simulink model "TCSC_original"  (R2024a)
settings: Solver=FixedStepAuto  StartTime=0.0  StopTime=5  FixedStep=Ts  MaxStep=2*Ts  RelTol=1e-4  AbsTol=1e-4
PreLoadFcn:
  | Ts=50e-6;
undefined symbols (not defined in the file or in its folder): DiscIntNeverNeededParam, find_system
libraries: spsEdgeDetectorLib x12, spsSampleandHoldLib x6, spsSeriesRLCBranchLib x6, spsThyristorLib x6, spsVoltageMeasurementLib x4, spsBistableLib x3, spsMeanVariableFrequencyLib x3, spsSecondOrderFilterLib x3, spsBreakerLib x3, spsCurrentMeasurementLib x3, spsThreePhaseVIMeasurementLib x2, spsGroundLib x2
(part 1 of 2)
settings Model: Creator=The MathWorks, Inc.  LastModifiedBy=E370_
settings SolverCC: AutoScaleAbsTol=off  AlgebraicLoopSolver=TrustRegion
settings DataIOCC: SaveFormat=StructureWithTime  SaveOutput=off  SignalLogging=off  DSMLogging=off  SaveTime=off  ReturnWorkspaceOutputs=off  SignalLoggingName=sigsOut
settings OptimizationCC: BooleanDataType=off  ExpressionDepthLimit=2147483647  InitFltsAndDblsToZero=on  LifeSpan=inf
settings DebuggingCC: SaveWithParameterizedLinksMsg=none  UnderspecifiedInitializationDetection=Classic  MergeDetectMultiDrivingBlocksExec=none  CheckExecutionContextPreStartOutputMsg=on  SignalResolutionControl=TryResolveAllWithWarning  MultiTaskDSMMsg=warning  MultiTaskCondExecSysMsg=none  FcnCallInpInsideContextMsg=warning  UnconnectedInputMsg=warning  UnconnectedOutputMsg=warning  UnconnectedLineMsg=warning  StateNameClashWarn=warning  SFUnexpectedBacktrackingDiag=warning  SFNoUnconditionalDefaultTransitionDiag=warning  SFExecutionAtInitializationDiag=none  ArithmeticOperatorsInVariantConditions=warning
settings HardwareCC: ProdBitPerPointer=32  ProdBitPerSizeT=32  ProdBitPerPtrDiffT=32  ProdLargestAtomicFloat=None  ProdIntDivRoundTo=Undefined  ProdEndianess=Unspecified  ProdWordSize=32  ProdHWDeviceType=32-bit Generic  TargetUnknown=on
settings ModelReferenceCC: EnableRefExpFcnMdlSchedulingChecks=on  PropagateSignalLabelsOutOfModel=off
settings SFSimCC: SimUseLocalCustomCode=off  CustomCodeUndefinedFunction=UseInterfaceOnly
settings RTWCC: RTWUseLocalCustomCode=off  GPUComputeCapability=3.5  DLArmComputeVersion=19.05
settings CodeAppCC: StateflowObjectComments=on
settings GRTTargetCC: TargetFcnLib=ansi_tfl_tmw.mat  TargetLangStandard=C89/C90 (ANSI)  CombineOutputUpdateFcns=off  GRTInterface=on
settings ConfigComp: CovMetricSettings=dw  CovSaveCumulativeToWorkspaceVar=on  CovSaveSingleToWorkspaceVar=on  CovExternalEMLEnable=off  CovSFcnEnable=off
settings SimscapeCC: SimscapeNormalizeSystem=off

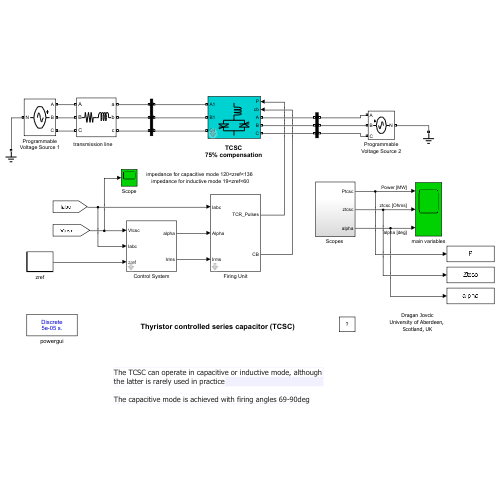
[thumbnail: Simulink's stored preview of the top-level diagram]
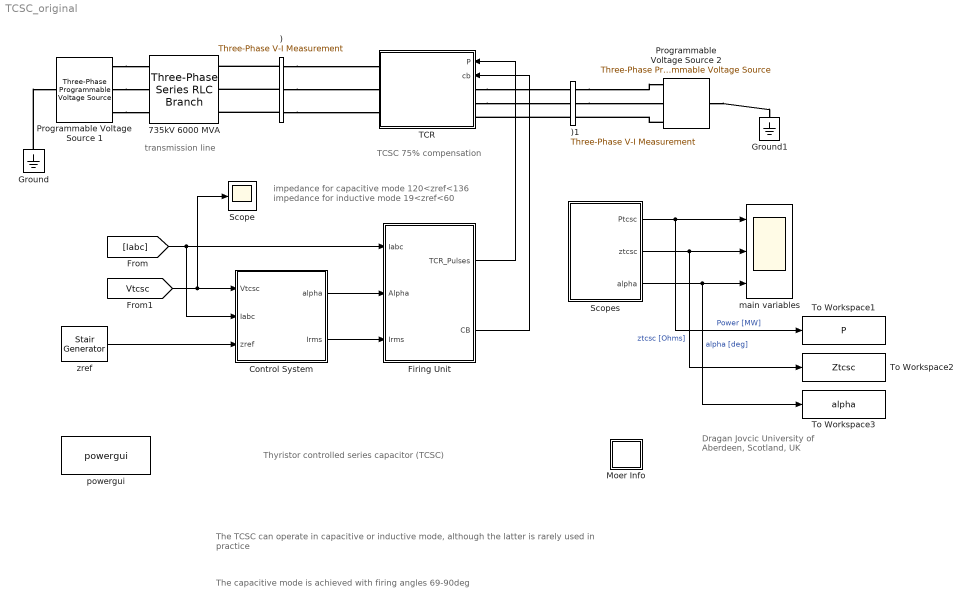
== system TCSC_original ==
  note: The TCSC can operate in capacitive or inductive mode, although the latter is rarely used in practice
  note: The capacitive mode is achieved with firing angles 69-90deg
  note: Thyristor controlled series capacitor (TCSC)
  note: TCSC
      | 75% compensation
  note: transmission line
  note: Dragan Jovcic
      | University of Aberdeen,
      | Scotland, UK
  note: impedance for capacitive mode 120<zref<136
      |  impedance for inductive mode 19<zref<60
  ) : spsThreePhaseVIMeasurementLib/Three-Phase V-I Measurement  VoltageMeasurement=phase-to-ground  SetLabelV=on  LabelV=Vabc1  Vpu=off  VpuLL=off  CurrentMeasurement=yes  SetLabelI=on  LabelI=Iabc  Ipu=off  Pbase=400e6  Vbase=477.8e3  OutputType=Magnitude  PhasorSimulation=off  PSBequivalent=0
  )1 : spsThreePhaseVIMeasurementLib/Three-Phase V-I Measurement  VoltageMeasurement=phase-to-ground  SetLabelV=on  LabelV=Vabc2  Vpu=off  VpuLL=off  CurrentMeasurement=yes  SetLabelI=on  LabelI=Iabc2  Ipu=off  Pbase=100e6  Vbase=477.8e3  OutputType=Magnitude  PhasorSimulation=off  PSBequivalent=0
  "735kV 6000 MVA " : spsThreePhaseSeriesRLCBranchLib/Three-Phase Series RLC Branch  LConnTagsString=A|B|C  RConnTagsString=A|B|C  BranchType=RL  Resistance=6.0852  Inductance=0.4323  Capacitance=[]  Measurements=None
  Control System : Subsystem  mask(TCSC control system){ParI=[0 60], mode=capacitive, Ts=Ts, man_alpha=78}
      mask prompts: ParI "Initial input: [Phase (degree) Freq (Hz) ]"; mode "Operating mode"; Ts "Sample time:"; man_alpha "Manual alpha [deg] (used in manual mode)"
      mask init:
      | Phase_Init=ParI(1);
      | Freq_Init=ParI(2);
      mask Help: This block includes system level controllers for TCSC. It determines the TCSC firing angle using the reference impedance and the measured voltage and current. The TCSC controller can operate in constant inductive/capacitive/firing angle mode.
      mask TypeOptions mode: inductive  | capacitive | manual alpha
  Firing Unit : Subsystem  mask(TCSC Firing Unit){FiringMode=Synchronized, Nstep=0, ParInit=[0 60], Ts=Ts}
      mask prompts: FiringMode "Firing mode"; Nstep "Total delay (in number of time step)"; ParInit "Initial phase and frequency of input: [ Phase (degree)  Freq (Hz) ]"; Ts "Sample time:"
      mask init:
      | PhaseInit=ParInit(1);
      | FreqInit=ParInit(2);
      mask Help: This block determines the firing signals for TCSC thyristors. It uses the firing angle alpha as the input. The line current is used as the synchronising signal.
      mask TypeOptions FiringMode: Synchronized | Continuous
  Ground : spsGroundLib/Ground  LConnTagsString=a
  Ground1 : spsGroundLib/Ground  LConnTagsString=a
  Moer Info : Subsystem
      settings: OpenFcn="showExample(\"simscapeelectricalsps/ThyristorControlledSeriesCapacitorExample\")"
      mask Display: disp('?')
  Programmable Voltage Source 1 : spsThreePhaseProgrammableVoltageSourceLib/Three-Phase Programmable Voltage Source  PositiveSequence="[1.00*539e3 0  60]"  VariationEntity=Amplitude  VariationType=Table of time-amplitude pairs  VariationTypeAlt=Step  VariationStep=-0.3  VariationRate=0.5  VariationMagnitude=0.4  VariationFrequency=2  VariationTiming=[0.1 1.2]  VariationPhaseA=off  Amplitudes=[1.0 0.96 1.0 ]  TimeValues=[0 3.3 3.8 ]  HarmonicGeneration=off  HarmonicA=[3 0.2 -25 0]  HarmonicB="[2 0.15  35 2]"  Timing="[0.1  0.6]"  BusType=swing  Pref=0  Qref=0  Qmin=-inf  Qmax=inf
  Programmable Voltage Source 2 : spsThreePhaseProgrammableVoltageSourceLib/Three-Phase Programmable Voltage Source  PositiveSequence="[1.0*477.8e3 -3.813  60]"  VariationEntity=Amplitude  VariationType=Table of time-amplitude pairs  VariationTypeAlt=Step  VariationStep=-0.3  VariationRate=0.5  VariationMagnitude=0.4  VariationFrequency=2  VariationTiming=[0.1 1.2]  VariationPhaseA=off  Amplitudes=[1]  TimeValues=[0]  HarmonicGeneration=off  HarmonicA=[3 0.2 -25 0]  HarmonicB="[2 0.15  35 2]"  Timing="[0.1  0.6]"  BusType=swing  Pref=0  Qref=0  Qmin=-inf  Qmax=inf
  Scope : Scope
  "Scopes " : Subsystem
  TCR : Subsystem  LoadFcn=find_system(gcs,'FollowLinks', 'on', 'LookUnderMasks', 'all');  mask(TCSC model){Ltcr=0.043, Ctcsc=21.977e-6, Q=500, ParS=[5000 50e-9], ParT=[1e-2  0]}
      mask prompts: Ltcr "TCR Inductance (H) :"; Ctcsc "TCSC capacitance (F)"; Q "Quality factor:"; ParS "Thyristor snubber: [ R (ohm)   C (F)  ]"; ParT "Thyristor data: [ Ron (ohm)   Vf (volt) ]"
      mask init:
      | Rtcr=(2*pi*60) * Ltcr / Q;
      | Rsnub=ParS(1);
      | Csnub=ParS(2);
      | Ron=ParT(1);
      | Vf=ParT(2);
      mask Help:
      | This block is main circuit of a TCSC. The TCSC includes a series TCR and a series capacitor in each phase.
      | The model parameters are L=0.043 and C=21.977uF giving the natural resonance at 163Hz. The resonant firing angle (60Hz system) is around 58deg.
      mask Display:
      | plot(0,0);plot(125,220)
      | plot([62 62 37 37 49 25 37],[15 39 39 58 76 76 58])
      | plot([62 87 87 99 87 75 87],[39 39 58 58 76 58 58])
      | plot([25 49],[58 58]);plot([37 25],[58 49])
      | plot([75 99],[76 76]);plot([87 99],[76 85])
      | plot([37 37 87 87],[76 95 95 76])
      | plot([62 62],[95 122]);plot([62 62],[164 186])
      | plot([62 72 78 79 78 72 62],[122 123 125 129 133 135 136])
      | plot([62 72 78 79 78 72 62],14+[122 123 125 129 133 135 136])
      | plot([62 72 78 79 78 72 62],28+[122 123 125 129 133 135 136])
  To Workspace1 : ToWorkspace  VariableName=P  SaveFormat=Timeseries  SampleTime=-1
  To Workspace2 : ToWorkspace  VariableName=Ztcsc  SaveFormat=Timeseries  SampleTime=-1
  To Workspace3 : ToWorkspace  VariableName=alpha  SaveFormat=Timeseries  SampleTime=-1
  main variables : Scope  NumInputPorts=3
  powergui : spspowerguiLib/powergui  Priority=2  SimulationMode=Discrete  SampleTime=Ts  frequency=60  Iterations=50  frequencyindice=60  Pbase=100e6  ErrMax=1e-4  UnitsV=kV  UnitsW=MW  buscounter=0  FunctionMessages=off  echomessages=off  EnableUseOfTLC=off  CurrentSourceSwitches=off  DisableSnubberDevices=off  DisableRonSwitches=off  DisableVfSwitches=off  DisplayEquations=off  AutomaticDiscreteSolvers=off  SolverType=Tustin/Backward Euler (TBE)  Interpol=off  ExternalGateDelay=off  methode=off  Ts=0  x0status=blocks  SPID=off  SwTol=0  HookPort=off  NonlinearTolerance=0  nMaxIteration=15  ContinueOnMaxIteration=off  RestoreLinks=warning  ResistiveCurrentMeasurement=off  Frange=[0:2:500]  Ylog=off  Xlog=on  ShowGrid=off  save=off  variable=ZData  structure=0  ZoomFFT=on  StartTime=0.0  cycles=1  DisplayStyle=1  fundamental=60  FreqAxis=off  MaxFrequency=1000  frequencyindicesteady=1  RmsSteady=2  display=off
  zref : spsStairGeneratorLib/Stair Generator  t="[ 0  2.5   5 ]"  e="[1.0 0.95  0.95 ]*128"  Ts=Ts
  wires:
  "Scopes "/1(Ptcsc) -> To Workspace1/1, main variables/1  "Power [MW]"
  "Scopes "/2(ztcsc) -> To Workspace2/1, main variables/2  "ztcsc [Ohms]"
  [Iabc] -> Control System/2(Iabc), Firing Unit/1(Iabc)
  Firing Unit/1(TCR_Pulses) -> TCR/1(P)
  Control System/1(alpha) -> Firing Unit/2(Alpha)
  Control System/2(Irms) -> Firing Unit/3(Irms)
  Firing Unit/2(CB) -> TCR/2(cb)
  "Scopes "/3(alpha) -> To Workspace3/1, main variables/3  "alpha [deg]"
  [Vtcsc] -> Scope/1, Control System/1(Vtcsc)
  zref/1 -> Control System/3(zref)
  connections:
  Ground/LConn1 -- Programmable Voltage Source 1/LConn1
  )/LConn1 -- "735kV 6000 MVA "/RConn1
  )/LConn2 -- "735kV 6000 MVA "/RConn2
  Programmable Voltage Source 1/RConn2 -- "735kV 6000 MVA "/LConn2
  Programmable Voltage Source 1/RConn3 -- "735kV 6000 MVA "/LConn3
  Programmable Voltage Source 1/RConn1 -- "735kV 6000 MVA "/LConn1
  )/LConn3 -- "735kV 6000 MVA "/RConn3
  Programmable Voltage Source 2/LConn1 -- Ground1/LConn1
  Programmable Voltage Source 2/RConn3 -- )1/RConn3
  )1/RConn2 -- Programmable Voltage Source 2/RConn2
  )1/RConn1 -- Programmable Voltage Source 2/RConn1
  )/RConn3 -- TCR/RConn3
  )/RConn2 -- TCR/RConn2
  )/RConn1 -- TCR/RConn1
  TCR/LConn1 -- )1/LConn1
  TCR/LConn2 -- )1/LConn2
  )1/LConn3 -- TCR/LConn3

== system TCSC_original/Control System ==
  note: Dragan Jovcic
      | University of Aberdeen,
      | Scotland, UK
  Vtcsc : Inport  PortDimensions=3
  Iabc : Inport  Port=2  PortDimensions=3
  zref : Inport  Port=3  PortDimensions=1
  Add1 : Sum  Inputs=+-
  Controller capacitive mode : Subsystem  mask(Controller in capacitive mode){kpc=0.8, kic=4.6}
      mask prompts: kpc "proportional gain"; kic "integral gain"
      mask init:
      | power_initmask();
      settings: OpenFcn=power_openblockproxy();
      mask Help: helpview(psbhelp)
  Controller inductive mode : Subsystem  mask(Controller in inductive mode){kpin=0.6, kiin=17}
      mask prompts: kpin "proportional gain"; kiin "integral gain"
      mask init:
      | power_initmask();
      settings: OpenFcn=power_openblockproxy();
      mask Help: helpview(psbhelp)
  Impedance calculation : Subsystem
  Switch1 : Switch  Threshold=2  SaturateOnIntegerOverflow=off  InputSameDT=off
  Switch2 : Switch  Threshold=3  SaturateOnIntegerOverflow=off  InputSameDT=off
  manual alpha : Subsystem
  operating mode : Constant  Value=mode
  reference impedance1 : Constant
  alpha : Outport  VectorParamsAs1DForOutWhenUnconnected=off
  Irms : Outport  Port=2  VectorParamsAs1DForOutWhenUnconnected=off
  tag scope: alpha=global, mode1=global, mode=global
  wires:
  Switch2/1 -> alpha/1, [alpha]
  Controller capacitive mode/1(alpha capacitive) -> Switch1/1
  Controller inductive mode/1(alpha inductive) -> Switch1/3
  operating mode/1 -> Switch1/2, Switch2/2, [mode], Add1/1
  manual alpha/1(alpha manual) -> Switch2/1
  Impedance calculation/1(impedance) -> Controller capacitive mode/1(zmeasured), Controller inductive mode/1(zmeasured)
  Impedance calculation/2(Irms) -> Irms/1
  Switch1/1 -> Switch2/3
  Add1/1 -> [mode1]
  reference impedance1/1 -> Add1/2
  zref/1 -> Controller capacitive mode/2(zreference), Controller inductive mode/2(zreference)
  Vtcsc/1 -> Impedance calculation/1(Vtcsca)
  Iabc/1 -> Impedance calculation/2(Iabc)

== system TCSC_original/Firing Unit ==
  note: TCSC bypassed for first 0.5s
  Iabc : Inport  PortDimensions=3
  Alpha : Inport  Port=2  PortDimensions=1
  Irms : Inport  Port=3  PortDimensions=1
  Clock : Clock
  Constant1 : Constant
  Constant4 : Constant  Value=0
  Demux : Demux  Outputs=3
      settings: DisplayOption=none
  Firing Unit A phase : Subsystem  mask{FiringMode=FiringMode, Nstep=Nstep, ParInit=[PhaseInit FreqInit], Ts=Ts}
      mask prompts: FiringMode "Firing Mode (1=Synchronized, 2=Continuous)"; Nstep "Total delay (in number of time step)"; ParInit "Initial phase and frequency of input: [ Phase (degree)  Freq (Hz) ]"; Ts "Sample time:"
      mask init:
      | PhaseInit=ParInit(1);
      | FreqInit=ParInit(2);
  Firing Unit B phase : Subsystem  mask{FiringMode=FiringMode, Nstep=Nstep, ParInit=[PhaseInit-120  FreqInit], Ts=Ts}
      mask prompts: FiringMode "Firing Mode (1=Synchronized, 2=Continuous)"; Nstep "Total delay (in number of time step)"; ParInit "Initial phase and frequency of input: [ Phase (degree)  Freq (Hz) ]"; Ts "Sample time:"
      mask init:
      | PhaseInit=ParInit(1);
      | FreqInit=ParInit(2);
  Firing Unit C phase : Subsystem  mask{FiringMode=FiringMode, Nstep=Nstep, ParInit=[PhaseInit+120  FreqInit], Ts=Ts}
      mask prompts: FiringMode "Firing Mode (1=Synchronized, 2=Continuous)"; Nstep "Total delay (in number of time step)"; ParInit "Initial phase and frequency of input: [ Phase (degree)  Freq (Hz) ]"; Ts "Sample time:"
      mask init:
      | PhaseInit=ParInit(1);
      | FreqInit=ParInit(2);
  Mux : Mux  Inputs=6
  Switch1 : Switch  Threshold=0.5  SaturateOnIntegerOverflow=off  InputSameDT=off
  current p.u. : Subsystem
  TCR_Pulses : Outport  VectorParamsAs1DForOutWhenUnconnected=off
  CB : Outport  Port=2  VectorParamsAs1DForOutWhenUnconnected=off
  tag scope: CB=global, TCR_pulses=global
  wires:
  Demux/1 -> Firing Unit A phase/1(Iabc)
  Demux/2 -> Firing Unit B phase/1(Iabc)
  Demux/3 -> Firing Unit C phase/1(Iabc)
  Firing Unit A phase/1(TCR +) -> Mux/1
  Firing Unit B phase/1(TCR +) -> Mux/3
  Firing Unit B phase/2(TCR -) -> Mux/4
  Firing Unit C phase/1(TCR +) -> Mux/5
  Firing Unit C phase/2(TCR -) -> Mux/6
  Mux/1 -> TCR_Pulses/1, [TCR_pulses]
  Irms/1 -> current p.u./3(Irms)
  Constant4/1 -> Switch1/1
  Constant1/1 -> Switch1/3
  Clock/1 -> Switch1/2
  Switch1/1 -> CB/1, [CB]
  current p.u./1("Iabc_pu ") -> Demux/1
  Iabc/1 -> current p.u./1(Iabc)
  Alpha/1 -> current p.u./2(alpha), Firing Unit A phase/2(Alpha), Firing Unit C phase/2(Alpha), Firing Unit B phase/2(Alpha)
  Firing Unit A phase/2(TCR -) -> Mux/2

== system TCSC_original/Moer Info ==

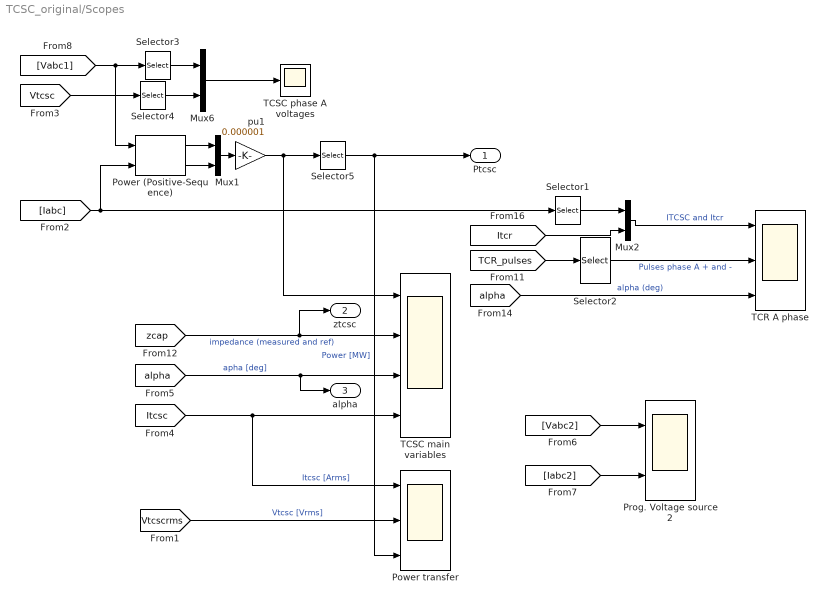
== system TCSC_original/Scopes  ==
  Mux1 : Mux  Inputs=2
  Mux2 : Mux  Inputs=2
  Mux6 : Mux  Inputs=2
  Power (Positive-Sequence) : spsPowerPositiveSequenceLib/Power (Positive-Sequence)  Freq=60  Vinit=[1 0]  Iinit=[0.05 90]  Ts=Ts
  Power transfer : Scope  NumInputPorts=3
  Prog. Voltage source 2 : Scope  NumInputPorts=2
  Selector1 : Selector  InputPortWidth=3  IndexOptions=Index vector (dialog)  Indices=1  OutputSizes=1
  Selector2 : Selector  InputPortWidth=6  IndexOptions=Index vector (dialog)  Indices=[1 2]  OutputSizes=1
  Selector3 : Selector  InputPortWidth=3  IndexOptions=Index vector (dialog)  Indices=1  OutputSizes=1
  Selector4 : Selector  InputPortWidth=3  IndexOptions=Index vector (dialog)  Indices=1  OutputSizes=1
  Selector5 : Selector  InputPortWidth=2  IndexOptions=Index vector (dialog)  Indices=1  OutputSizes=1
  TCR A phase : Scope  NumInputPorts=3
  TCSC main variables : Scope  NumInputPorts=4
  TCSC phase A voltages : Scope
  pu1 : Gain  Gain=0.000001  SaturateOnIntegerOverflow=on  OutDataTypeStr=Inherit: Same as input  ParamDataTypeStr=Inherit: Same as input
  Ptcsc : Outport  VectorParamsAs1DForOutWhenUnconnected=off
  ztcsc : Outport  Port=2  VectorParamsAs1DForOutWhenUnconnected=off
  alpha : Outport  Port=3  VectorParamsAs1DForOutWhenUnconnected=off
  wires:
  [Vabc1] -> Power (Positive-Sequence)/1, Selector3/1
  [alpha] -> TCSC main variables/3, alpha/1  "apha [deg]"
  [TCR_pulses] -> Selector2/1
  Selector2/1 -> TCR A phase/2  "Pulses phase A + and -"
  [alpha] -> TCR A phase/3  "alpha (deg)"
  [Itcr] -> Mux2/2
  Mux2/1 -> TCR A phase/1  "ITCSC and Itcr"
  Selector3/1 -> Mux6/1
  [Itcsc] -> TCSC main variables/4, Power transfer/1  "Itcsc [Arms]"
  [zcap] -> TCSC main variables/2, ztcsc/1  "impedance (measured and ref)"
  pu1/1 -> TCSC main variables/1, Selector5/1
  [Vtcscrms] -> Power transfer/2  "Vtcsc [Vrms]"
  [Iabc] -> Power (Positive-Sequence)/2, Selector1/1
  Selector1/1 -> Mux2/1
  Mux6/1 -> TCSC phase A voltages/1
  Selector4/1 -> Mux6/2
  [Vtcsc] -> Selector4/1
  [Iabc2] -> Prog. Voltage source 2/2
  [Vabc2] -> Prog. Voltage source 2/1
  Power (Positive-Sequence)/1 -> Mux1/1
  Power (Positive-Sequence)/2 -> Mux1/2
  Mux1/1 -> pu1/1
  Selector5/1 -> Power transfer/3, Ptcsc/1  "Power [MW]"

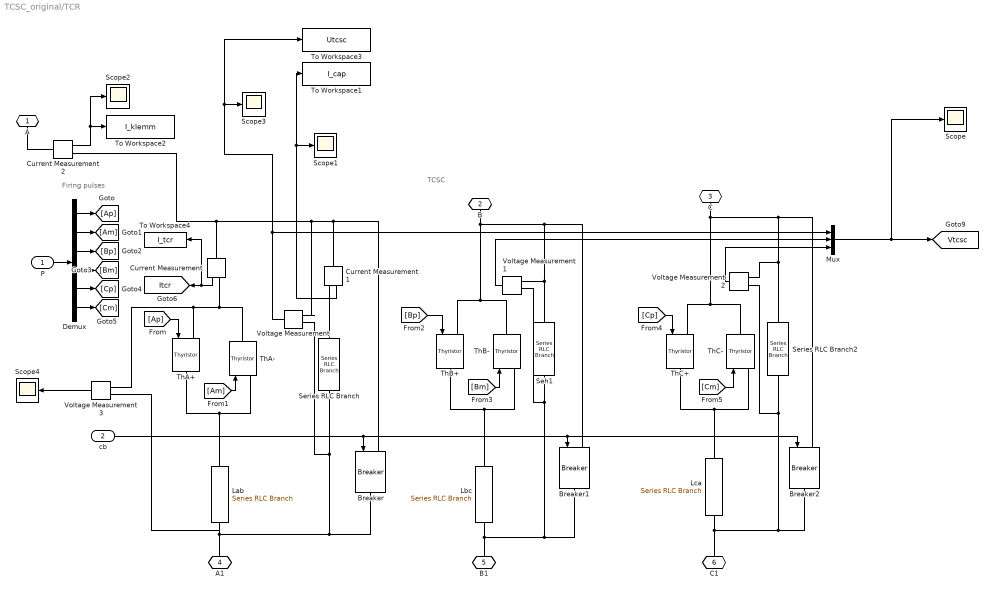
== system TCSC_original/TCR ==
  note: Firing pulses
  note: TCSC
  P : Inport  PortDimensions=6
  cb : Inport  Port=2  PortDimensions=1
  Breaker : spsBreakerLib/Breaker  InitialState=0  SwitchingTimes="[ 1/60  5/60 ]"  External=on  BreakerResistance=0.01  SnubberResistance=1e6  SnubberCapacitance=inf  Measurements=None  MoreParameters=off  NoBreakLoop=off
  Breaker1 : spsBreakerLib/Breaker  InitialState=0  SwitchingTimes="[ 1/60  5/60 ]"  External=on  BreakerResistance=0.01  SnubberResistance=1e6  SnubberCapacitance=inf  Measurements=None  MoreParameters=off  NoBreakLoop=off
  Breaker2 : spsBreakerLib/Breaker  InitialState=0  SwitchingTimes="[ 1/60  5/60 ]"  External=on  BreakerResistance=0.01  SnubberResistance=1e6  SnubberCapacitance=inf  Measurements=None  MoreParameters=off  NoBreakLoop=off
  Current Measurement : spsCurrentMeasurementLib/Current Measurement  PhasorSimulation=off  OutputType=Complex  PSBequivalent=0
  Current Measurement1 : spsCurrentMeasurementLib/Current Measurement  PhasorSimulation=off  OutputType=Complex  PSBequivalent=0
  Current Measurement2 : spsCurrentMeasurementLib/Current Measurement  PhasorSimulation=off  OutputType=Complex  PSBequivalent=0
  Demux : Demux  Outputs=6
      settings: DisplayOption=none
  Lab : spsSeriesRLCBranchLib/Series RLC Branch  LConnTagsString=__new0  RConnTagsString=__new0  BranchType=RL  Resistance=Rtcr  Inductance=Ltcr  SetiL0=off  InitialCurrent=0  Capacitance=[]  Setx0=off  InitialVoltage=0  Measurements=Branch current
  Lbc : spsSeriesRLCBranchLib/Series RLC Branch  LConnTagsString=__new0  RConnTagsString=__new0  BranchType=RL  Resistance=Rtcr  Inductance=Ltcr  SetiL0=off  InitialCurrent=0  Capacitance=[]  Setx0=off  InitialVoltage=0  Measurements=None
  Lca : spsSeriesRLCBranchLib/Series RLC Branch  LConnTagsString=__new0  RConnTagsString=__new0  BranchType=RL  Resistance=Rtcr  Inductance=Ltcr  SetiL0=off  InitialCurrent=0  Capacitance=[]  Setx0=off  InitialVoltage=0  Measurements=None
  Mux : Mux  Inputs=3
  Scope{,1..4} (5 alike) : Scope
  Seh1 : spsSeriesRLCBranchLib/Series RLC Branch  LConnTagsString=__new0  RConnTagsString=__new0  BranchType=C  Resistance=[]  Inductance=[]  SetiL0=off  InitialCurrent=0  Capacitance=Ctcsc  Setx0=off  InitialVoltage=0  Measurements=None
  Series RLC Branch : spsSeriesRLCBranchLib/Series RLC Branch  LConnTagsString=__new0  RConnTagsString=__new0  BranchType=C  Resistance=[]  Inductance=[]  SetiL0=off  InitialCurrent=0  Capacitance=Ctcsc  Setx0=off  InitialVoltage=0  Measurements=None
  Series RLC Branch2 : spsSeriesRLCBranchLib/Series RLC Branch  LConnTagsString=__new0  RConnTagsString=__new0  BranchType=C  Resistance=[]  Inductance=[]  SetiL0=off  InitialCurrent=0  Capacitance=Ctcsc  Setx0=off  InitialVoltage=0  Measurements=None
  ThA+ : spsThyristorLib/Thyristor  Ron=Ron  Lon=0  Vf=Vf  IC=0  Rs=Rsnub  Cs=Csnub  Measurements=off
      settings: AttributesFormatString=\n
  ThA- : spsThyristorLib/Thyristor  Ron=Ron  Lon=0  Vf=Vf  IC=0  Rs=Rsnub  Cs=Csnub  Measurements=off
      settings: AttributesFormatString=\n
  ThB+ : spsThyristorLib/Thyristor  Ron=Ron  Lon=0  Vf=Vf  IC=0  Rs=Rsnub  Cs=Csnub  Measurements=off
      settings: AttributesFormatString=\n
  ThB- : spsThyristorLib/Thyristor  Ron=Ron  Lon=0  Vf=Vf  IC=0  Rs=Rsnub  Cs=Csnub  Measurements=off
      settings: AttributesFormatString=\n
  ThC+ : spsThyristorLib/Thyristor  Ron=Ron  Lon=0  Vf=Vf  IC=0  Rs=Rsnub  Cs=Csnub  Measurements=off
      settings: AttributesFormatString=\n
  ThC- : spsThyristorLib/Thyristor  Ron=Ron  Lon=0  Vf=Vf  IC=0  Rs=Rsnub  Cs=Csnub  Measurements=off
      settings: AttributesFormatString=\n
  To Workspace1 : ToWorkspace  VariableName=I_cap  SaveFormat=Timeseries  SampleTime=-1
  To Workspace2 : ToWorkspace  VariableName=I_klemm  SaveFormat=Timeseries  SampleTime=-1
  To Workspace3 : ToWorkspace  VariableName=Utcsc  SaveFormat=Timeseries  SampleTime=-1
  To Workspace4 : ToWorkspace  VariableName=I_tcr  SaveFormat=Timeseries  SampleTime=-1
  Voltage Measurement{,1..3} (4 alike) : spsVoltageMeasurementLib/Voltage Measurement  PhasorSimulation=off  OutputType=Complex  PSBequivalent=0
  A : PMIOPort  Side=Left
  B : PMIOPort  Port=2  Side=Left
  C : PMIOPort  Port=3  Side=Left
  A1 : PMIOPort  Port=4  Side=Right
  B1 : PMIOPort  Port=5  Side=Right
  C1 : PMIOPort  Port=6  Side=Right
  tag scope: Itcr=global, Vtcsc=global
  wires:
  P/1 -> Demux/1
  Demux/1 -> [Ap]
  Demux/2 -> [Am]
  Demux/3 -> [Bp]
  Demux/4 -> [Bm]
  Demux/5 -> [Cp]
  [Cp] -> ThC+/1
  [Cm] -> ThC-/1
  Demux/6 -> [Cm]
  [Bm] -> ThB-/1
  [Bp] -> ThB+/1
  [Am] -> ThA-/1
  [Ap] -> ThA+/1
  Current Measurement/1 -> To Workspace4/1, [Itcr]
  Voltage Measurement/1 -> Scope3/1, To Workspace3/1, Mux/1
  cb/1 -> Breaker/1, Breaker1/1, Breaker2/1
  Voltage Measurement1/1 -> Mux/2
  Mux/1 -> Scope/1, [Vtcsc]
  Voltage Measurement2/1 -> Mux/3
  Current Measurement1/1 -> To Workspace1/1, Scope1/1
  Voltage Measurement3/1 -> Scope4/1
  Current Measurement2/1 -> Scope2/1, To Workspace2/1
  connections:
  ThA-/LConn1 -- Lab/LConn1 -- ThA+/RConn1
  Current Measurement1/RConn1 -- Series RLC Branch/LConn1
  ThB-/LConn1 -- Lbc/LConn1 -- ThB+/RConn1
  Seh1/LConn1 -- ThB-/RConn1 -- ThB+/LConn1 -- B/RConn1 -- Breaker1/LConn1 -- Voltage Measurement1/LConn1
  ThC-/LConn1 -- ThC+/RConn1 -- Lca/LConn1
  Series RLC Branch2/LConn1 -- ThC-/RConn1 -- ThC+/LConn1 -- C/RConn1 -- Breaker2/LConn1 -- Voltage Measurement2/LConn1
  Voltage Measurement/LConn2 -- Series RLC Branch/RConn1 -- A1/RConn1 -- Voltage Measurement3/LConn1 -- Lab/RConn1 -- Breaker/RConn1
  Lbc/RConn1 -- B1/RConn1 -- Breaker1/RConn1 -- Seh1/RConn1 -- Voltage Measurement1/LConn2
  Series RLC Branch2/RConn1 -- Lca/RConn1 -- C1/RConn1 -- Breaker2/RConn1 -- Voltage Measurement2/LConn2
  ThA-/RConn1 -- Current Measurement/RConn1 -- Voltage Measurement3/LConn2 -- ThA+/LConn1
  Voltage Measurement/LConn1 -- Current Measurement2/RConn1 -- Current Measurement/LConn1 -- Current Measurement1/LConn1 -- Breaker/LConn1
  A/RConn1 -- Current Measurement2/LConn1

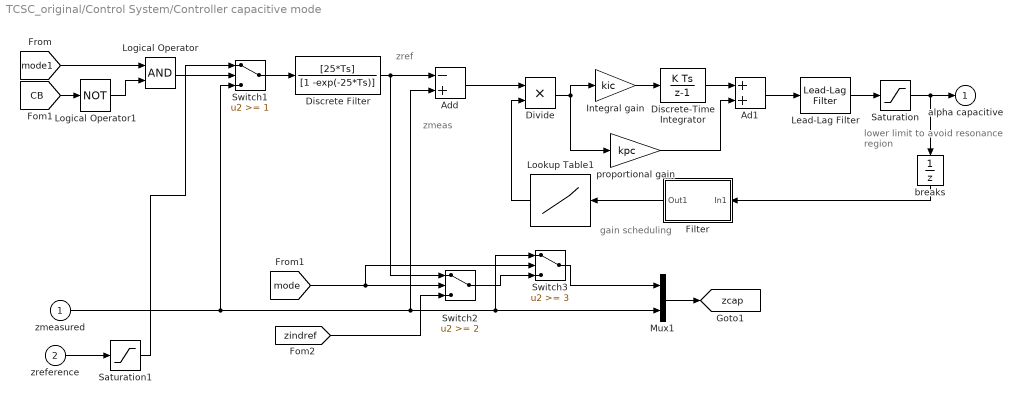
== system TCSC_original/Control System/Controller capacitive mode ==
  note: gain scheduling
  note: zref
  note: zmeas
  note: lower limit to
      | avoid resonance
      | region
  zmeasured : Inport
  zreference : Inport  Port=2
  Ad1 : Sum
  Add : Sum  Inputs=-+
  Discrete Filter : DiscreteFilter  Numerator=[25*Ts]  Denominator=[1 -exp(-25*Ts)]  SampleTime=Ts
  Discrete-Time Integrator : DiscreteIntegrator  InitialCondition=90  SampleTime=Ts  LimitOutput=on  UpperSaturationLimit=90  LowerSaturationLimit=69  ICPrevOutput=DiscIntNeverNeededParam  ICPrevScaledInput=DiscIntNeverNeededParam
  Divide : Product  Inputs=**
  Filter : Subsystem  TreatAsAtomicUnit=on
  Integral gain : Gain  Gain=kic
  Lead-Lag Filter : spsLeadLagFilterLib/Lead-Lag Filter  T1=0.05  T2=0.016  Vdc_Init=0  Ts=Ts
  Logical Operator : Logic  AllPortsSameDT=off  OutDataTypeStr=boolean
  Logical Operator1 : Logic  Operator=NOT  AllPortsSameDT=off  OutDataTypeStr=boolean
  Lookup Table1 : Lookup_n-D  NumberOfTableDimensions=1  BreakpointsForDimension1=[60 65 70 75 80 85 90]  BreakpointsForDimension2=[0 571.55 685.8 800.15 914.4 1028.8 1143.1 1257.4 1371.7 1486 1600.3 1714.6 1828.9 1943.2 2057.5 2171.8 2286.1 2400.5 2514.7 2629.1 2743.3 2857.7 2971.9 3086.3 3200.5 3314.9 3429.2]  Table=[0.3 0.67 0.83 0.96 0.98 0.994 1]  InternalRulePriority=Speed  RndMeth=Simplest
  Mux1 : Mux  Inputs=2
  Saturation : Saturate  UpperLimit=90  LowerLimit=69
  Saturation1 : Saturate  UpperLimit=136  LowerLimit=120.5
  Switch1 : Switch  Threshold=1  SaturateOnIntegerOverflow=off  InputSameDT=off
  Switch2 : Switch  Threshold=2  SaturateOnIntegerOverflow=off  InputSameDT=off
  Switch3 : Switch  Threshold=3  SaturateOnIntegerOverflow=off  InputSameDT=off
  breaks : UnitDelay  SampleTime=Ts  HasFrameUpgradeWarning=on
  proportional gain : Gain  Gain=kpc
  alpha capacitive : Outport  InitialOutput=0  VectorParamsAs1DForOutWhenUnconnected=off
  tag scope: zcap=global
  wires:
  zmeasured/1 -> Add/2, Mux1/2, Switch3/1, Switch1/3
  Saturation/1 -> alpha capacitive/1, breaks/1
  [CB] -> Logical Operator1/1
  Logical Operator1/1 -> Logical Operator/2
  Logical Operator/1 -> Switch1/2
  Saturation1/1 -> Switch1/1
  Switch1/1 -> Discrete Filter/1
  Discrete Filter/1 -> Add/1, Switch2/1
  Mux1/1 -> [zcap]
  zreference/1 -> Saturation1/1
  [mode] -> Switch2/2, Switch3/2
  [zindref] -> Switch2/3
  Lead-Lag Filter/1 -> Saturation/1
  Integral gain/1 -> Discrete-Time Integrator/1
  Discrete-Time Integrator/1 -> Ad1/1
  proportional gain/1 -> Ad1/2
  Divide/1 -> Integral gain/1, proportional gain/1
  Lookup Table1/1 -> Divide/2
  Add/1 -> Divide/1
  Filter/1(Out1) -> Lookup Table1/1
  Ad1/1 -> Lead-Lag Filter/1
  Switch3/1 -> Mux1/1
  Switch2/1 -> Switch3/3
  [mode1] -> Logical Operator/1
  breaks/1 -> Filter/1(In1)

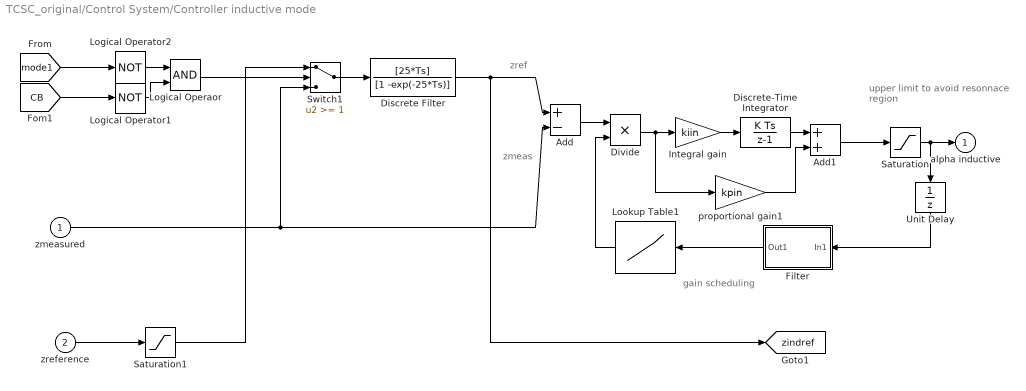
== system TCSC_original/Control System/Controller inductive mode ==
  note: gain scheduling
  note: upper limit to
      | avoid resonnace
      | region
  note: zref
  note: zmeas
  zmeasured : Inport
  zreference : Inport  Port=2
  Add : Sum  Inputs=+-
  Add1 : Sum
  Discrete Filter : DiscreteFilter  Numerator=[25*Ts]  Denominator=[1 -exp(-25*Ts)]  SampleTime=Ts
  Discrete-Time Integrator : DiscreteIntegrator  SampleTime=Ts  LimitOutput=on  UpperSaturationLimit=47  LowerSaturationLimit=0  ICPrevOutput=DiscIntNeverNeededParam  ICPrevScaledInput=DiscIntNeverNeededParam
  Divide : Product  Inputs=**
  Filter : Subsystem  TreatAsAtomicUnit=on
  Integral gain : Gain  Gain=kiin
  Logical Operaor : Logic  AllPortsSameDT=off  OutDataTypeStr=boolean
  Logical Operator1 : Logic  Operator=NOT  AllPortsSameDT=off  OutDataTypeStr=boolean
  Logical Operator2 : Logic  Operator=NOT  AllPortsSameDT=off  OutDataTypeStr=boolean
  Lookup Table1 : Lookup_n-D  NumberOfTableDimensions=1  BreakpointsForDimension1=[0 5 10 15 20 25 30 35 40 45 50 55]  BreakpointsForDimension2=[0 571.55 685.8 800.15 914.4 1028.8 1143.1 1257.4 1371.7 1486 1600.3 1714.6 1828.9 1943.2 2057.5 2171.8 2286.1 2400.5 2514.7 2629.1 2743.3 2857.7 2971.9 3086.3 3200.5 3314.9 3429.2]  Table="[1 0.95 0.9  0.875  0.86  0.76 0.68  0.58 0.44 0.3 0.15 0.04  ]"  InternalRulePriority=Speed  RndMeth=Simplest
  Saturation : Saturate  UpperLimit=47  LowerLimit=0
  Saturation1 : Saturate  UpperLimit=60  LowerLimit=19.3
  Switch1 : Switch  Threshold=1  SaturateOnIntegerOverflow=off  InputSameDT=off
  Unit Delay : UnitDelay  SampleTime=Ts  HasFrameUpgradeWarning=on
  proportional gain1 : Gain  Gain=kpin
  alpha inductive : Outport  InitialOutput=0  VectorParamsAs1DForOutWhenUnconnected=off
  tag scope: zindref=global
  wires:
  zmeasured/1 -> Add/2, Switch1/3
  Integral gain/1 -> Discrete-Time Integrator/1
  Discrete-Time Integrator/1 -> Add1/1
  proportional gain1/1 -> Add1/2
  Saturation/1 -> alpha inductive/1, Unit Delay/1
  [CB] -> Logical Operator1/1
  Logical Operator1/1 -> Logical Operaor/2
  Logical Operaor/1 -> Switch1/2
  Switch1/1 -> Discrete Filter/1
  Discrete Filter/1 -> Add/1, [zindref]
  zreference/1 -> Saturation1/1
  Saturation1/1 -> Switch1/1
  Divide/1 -> Integral gain/1, proportional gain1/1
  Add1/1 -> Saturation/1
  Filter/1(Out1) -> Lookup Table1/1
  Lookup Table1/1 -> Divide/2
  Add/1 -> Divide/1
  [mode1] -> Logical Operator2/1
  Logical Operator2/1 -> Logical Operaor/1
  Unit Delay/1 -> Filter/1(In1)

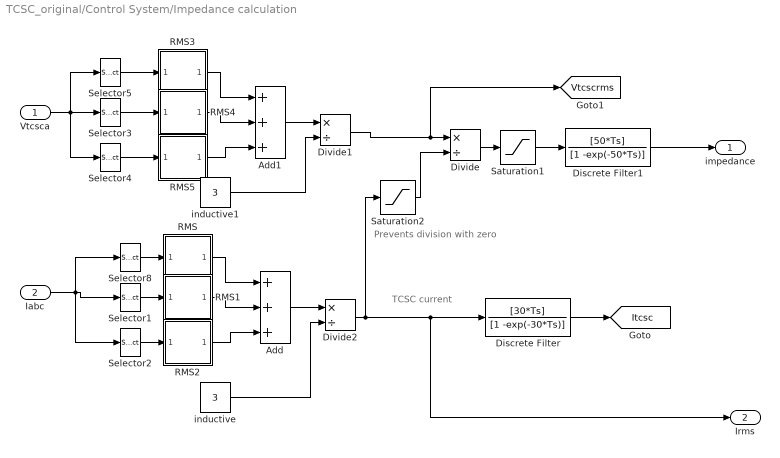
== system TCSC_original/Control System/Impedance calculation ==
  note: TCSC current
  note: Prevents division
      | with zero
  Vtcsca : Inport
  Iabc : Inport  Port=2
  Add : Sum  Inputs=+++
  Add1 : Sum  Inputs=+++
  Discrete Filter : DiscreteFilter  Numerator=[30*Ts]  Denominator=[1 -exp(-30*Ts)]  SampleTime=Ts
  Discrete Filter1 : DiscreteFilter  Numerator=[50*Ts]  Denominator=[1 -exp(-50*Ts)]  SampleTime=Ts
  Divide : Product  Inputs=*/
  Divide1 : Product  Inputs=*/
  Divide2 : Product  Inputs=*/
  RMS : Subsystem  mask(RMS){f1=60}
      mask prompts: f1 "Fundamental frequency (Hz):"
      mask help: This block measures the root mean square value of instantaneous current or voltage signal connected to the input of the block. The RMS value is calculated over a running window of one cycle of the specified fundamental frequency.
      mask init:
      | power_initmask();
      settings: OpenFcn=power_openblockproxy();
      mask Help: helpview(psbhelp)
  RMS1 : Subsystem  mask(RMS){f1=60}
      mask prompts: f1 "Fundamental frequency (Hz):"
      mask help: This block measures the root mean square value of instantaneous current or voltage signal connected to the input of the block. The RMS value is calculated over a running window of one cycle of the specified fundamental frequency.
      mask init:
      | power_initmask();
      settings: OpenFcn=power_openblockproxy();
      mask Help: helpview(psbhelp)
  RMS2 : Subsystem  mask(RMS){f1=60}
      mask prompts: f1 "Fundamental frequency (Hz):"
      mask help: This block measures the root mean square value of instantaneous current or voltage signal connected to the input of the block. The RMS value is calculated over a running window of one cycle of the specified fundamental frequency.
      mask init:
      | power_initmask();
      settings: OpenFcn=power_openblockproxy();
      mask Help: helpview(psbhelp)
  RMS3 : Subsystem  mask(RMS){f1=60}
      mask prompts: f1 "Fundamental frequency (Hz):"
      mask help: This block measures the root mean square value of instantaneous current or voltage signal connected to the input of the block. The RMS value is calculated over a running window of one cycle of the specified fundamental frequency.
      mask init:
      | power_initmask();
      settings: OpenFcn=power_openblockproxy();
      mask Help: helpview(psbhelp)
  RMS4 : Subsystem  mask(RMS){f1=60}
      mask prompts: f1 "Fundamental frequency (Hz):"
      mask help: This block measures the root mean square value of instantaneous current or voltage signal connected to the input of the block. The RMS value is calculated over a running window of one cycle of the specified fundamental frequency.
      mask init:
      | power_initmask();
      settings: OpenFcn=power_openblockproxy();
      mask Help: helpview(psbhelp)
  RMS5 : Subsystem  mask(RMS){f1=60}
      mask prompts: f1 "Fundamental frequency (Hz):"
      mask help: This block measures the root mean square value of instantaneous current or voltage signal connected to the input of the block. The RMS value is calculated over a running window of one cycle of the specified fundamental frequency.
      mask init:
      | power_initmask();
      settings: OpenFcn=power_openblockproxy();
      mask Help: helpview(psbhelp)
  Saturation1 : Saturate  UpperLimit=300  LowerLimit=10
  Saturation2 : Saturate  UpperLimit=1e10  LowerLimit=1e-10
  Selector1 : Selector  InputPortWidth=3  IndexOptions=Index vector (dialog)  Indices=2  OutputSizes=1
  Selector2 : Selector  InputPortWidth=3  IndexOptions=Index vector (dialog)  Indices=3  OutputSizes=1
  Selector3 : Selector  InputPortWidth=3  IndexOptions=Index vector (dialog)  Indices=2  OutputSizes=1
  Selector4 : Selector  InputPortWidth=3  IndexOptions=Index vector (dialog)  Indices=3  OutputSizes=1
  Selector5 : Selector  InputPortWidth=3  IndexOptions=Index vector (dialog)  Indices=1  OutputSizes=1
  Selector8 : Selector  InputPortWidth=3  IndexOptions=Index vector (dialog)  Indices=1  OutputSizes=1
  inductive : Constant  Value=3
  inductive1 : Constant  Value=3
  impedance : Outport  VectorParamsAs1DForOutWhenUnconnected=off
  Irms : Outport  Port=2  VectorParamsAs1DForOutWhenUnconnected=off
  tag scope: Itcsc=global, Vtcscrms=global
  wires:
  Divide1/1 -> Divide/1, [Vtcscrms]
  Divide/1 -> Saturation1/1
  Discrete Filter/1 -> [Itcsc]
  Selector8/1 -> RMS/1(signal)
  Discrete Filter1/1 -> impedance/1
  Selector1/1 -> RMS1/1(signal)
  Selector2/1 -> RMS2/1(signal)
  RMS/1(rms) -> Add/1
  RMS1/1(rms) -> Add/2
  RMS2/1(rms) -> Add/3
  Add/1 -> Divide2/1
  inductive/1 -> Divide2/2
  Divide2/1 -> Irms/1, Discrete Filter/1, Saturation2/1
  Iabc/1 -> Selector1/1, Selector8/1, Selector2/1
  RMS3/1(rms) -> Add1/1
  RMS4/1(rms) -> Add1/2
  RMS5/1(rms) -> Add1/3
  Add1/1 -> Divide1/1
  inductive1/1 -> Divide1/2
  Saturation1/1 -> Discrete Filter1/1
  Saturation2/1 -> Divide/2
  Vtcsca/1 -> Selector3/1, Selector5/1, Selector4/1
  Selector5/1 -> RMS3/1(signal)
  Selector3/1 -> RMS4/1(signal)
  Selector4/1 -> RMS5/1(signal)

== system TCSC_original/Control System/manual alpha ==
  Filter : Subsystem  TreatAsAtomicUnit=on
  Filter1 : Subsystem  TreatAsAtomicUnit=on
  Saturation : Saturate  UpperLimit=90  LowerLimit=68
  Saturation2 : Saturate  UpperLimit=49  LowerLimit=0
  Switch : Switch  Threshold=59  SaturateOnIntegerOverflow=off  InputSameDT=off
  Switch1 : Switch  Threshold=1  SaturateOnIntegerOverflow=off  InputSameDT=off
  Switch2 : Switch  Threshold=1  SaturateOnIntegerOverflow=off  InputSameDT=off
  initial alpha : Constant  Value=90
  initial alpha 1 : Constant  Value=0
  manual alpha : Constant  Value=man_alpha
  alpha manual : Outport  VectorParamsAs1DForOutWhenUnconnected=off
  wires:
  manual alpha/1 -> Switch/2, Switch2/3, Switch1/3
  Saturation/1 -> Switch/1
  Saturation2/1 -> Switch/3
  [CB] -> Switch2/2
  Switch/1 -> alpha manual/1
  initial alpha/1 -> Switch2/1
  Switch2/1 -> Filter/1(In1)
  Filter/1(Out1) -> Saturation/1
  [CB] -> Switch1/2
  Switch1/1 -> Filter1/1(In1)
  Filter1/1(Out1) -> Saturation2/1
  initial alpha 1/1 -> Switch1/1

== system TCSC_original/Firing Unit/Firing Unit A phase ==
  note: Generate square-wave synchronised with the line current.
      | For positive (Sync +) and negative (Sync -) transition
  note: PLL
      | sync on
      | pos. peak
      | of input
  note: Generate firing
      | pulse for TCR +
  note: Generate firing
      | pulse for TCR -
  note: Compute number
      | of samples per cycle
  note: Input
      | curent
  Iabc : Inport  PortDimensions=1
  Alpha : Inport  Port=2  PortDimensions=1
  BL2 : Subsystem
  BL3 : Subsystem
  Correction for delay : Gain  Gain=Nstep*Ts*2*pi  SaturateOnIntegerOverflow=on  OutDataTypeStr=Inherit: Same as input  ParamDataTypeStr=Inherit: Same as input
  Logical Operator2 : Logic  Operator=NOT  Inputs=3
  "PLL sync on positive peak " : Subsystem  mask(Discrete 1-phase PLL){Par_Init=[PhaseInit FreqInit], ParK=[50 500], Ts=Ts}
      mask prompts: Par_Init "Initial input:[ Phase(degrees)   Frequency(Hz) ]"; ParK "Regulator gains [ Kp  Ki ]"; Ts "Sample time:"
      mask help:
      | This Phase Locked Loop (PLL) system can be used  to synchronize on a variable frequency sinusoidal signal.
      |
      | Input 1: Normalized input signal V(pu)
      mask init:
      | Kp=ParK(1);
      | Ki=ParK(2);
      | Phase_Init=Par_Init(1);
      | Finit=Par_Init(2);
  Sum : Sum  InputSameDT=on  SaturateOnIntegerOverflow=on  OutDataTypeStr=Inherit: Same as first input
  TCR Pulse Generatorr : Subsystem  mask{Ts=Ts}
      mask prompts: Ts "Sample time:"
  TCR Pulse Generatorr1 : Subsystem  mask{Ts=Ts}
      mask prompts: Ts "Sample time:"
  Trigonometric Function6 : Trigonometry
  TCR + : Outport  VectorParamsAs1DForOutWhenUnconnected=off
  TCR - : Outport  Port=2  VectorParamsAs1DForOutWhenUnconnected=off
  wires:
  Logical Operator2/1 -> TCR Pulse Generatorr1/4(SqWave)
  TCR Pulse Generatorr/1(TCR +/-) -> TCR +/1
  BL3/1(SqWave) -> Logical Operator2/1, TCR Pulse Generatorr/4(SqWave)
  TCR Pulse Generatorr1/1(TCR +/-) -> TCR -/1
  BL3/2(Sync +) -> TCR Pulse Generatorr/3(Sync +/-)
  BL3/3(Sync -) -> TCR Pulse Generatorr1/3(Sync +/-)
  Alpha/1 -> TCR Pulse Generatorr/2(Alpha), TCR Pulse Generatorr1/2(Alpha)
  BL2/1(Ns/c) -> TCR Pulse Generatorr/1(Ns/c), TCR Pulse Generatorr1/1(Ns/c)
  "PLL sync on positive peak "/2(wt) -> Sum/2
  Sum/1 -> Trigonometric Function6/1
  Trigonometric Function6/1 -> BL3/2(sin(wt))
  Correction for delay/1 -> Sum/1
  "PLL sync on positive peak "/1(Freq) -> BL2/1(Freq), BL3/1(Freq), Correction for delay/1
  Iabc/1 -> "PLL sync on positive peak "/1(V(pu))

== system TCSC_original/Firing Unit/Firing Unit B phase ==
  note: Generate square-wave synchronised with the line current.
      | For positive (Sync +) and negative (Sync -) transition
  note: PLL
      | sync on
      | pos. peak
      | of input
  note: Generate firing
      | pulse for TCR +
  note: Generate firing
      | pulse for TCR -
  note: Compute number
      | of samples per cycle
  note: Input
      | curent
  Iabc : Inport  PortDimensions=1
  Alpha : Inport  Port=2  PortDimensions=1
  BL2 : Subsystem
  BL3 : Subsystem
  Correction for delay : Gain  Gain=Nstep*Ts*2*pi  SaturateOnIntegerOverflow=on  OutDataTypeStr=Inherit: Same as input  ParamDataTypeStr=Inherit: Same as input
  Logical Operator2 : Logic  Operator=NOT  Inputs=3
  "PLL sync on positive peak " : Subsystem  mask(Discrete 1-phase PLL){Par_Init=[PhaseInit FreqInit], ParK=[50 500], Ts=Ts}
      mask prompts: Par_Init "Initial input:[ Phase(degrees)   Frequency(Hz) ]"; ParK "Regulator gains [ Kp  Ki ]"; Ts "Sample time:"
      mask help:
      | This Phase Locked Loop (PLL) system can be used  to synchronize on a variable frequency sinusoidal signal.
      |
      | Input 1: Normalized input signal V(pu)
      mask init:
      | Kp=ParK(1);
      | Ki=ParK(2);
      | Phase_Init=Par_Init(1);
      | Finit=Par_Init(2);
  Sum : Sum  InputSameDT=on  SaturateOnIntegerOverflow=on  OutDataTypeStr=Inherit: Same as first input
  TCR Pulse Generatorr : Subsystem  mask{Ts=Ts}
      mask prompts: Ts "Sample time:"
  TCR Pulse Generatorr1 : Subsystem  mask{Ts=Ts}
      mask prompts: Ts "Sample time:"
  Trigonometric Function6 : Trigonometry
  TCR + : Outport  VectorParamsAs1DForOutWhenUnconnected=off
  TCR - : Outport  Port=2  VectorParamsAs1DForOutWhenUnconnected=off
  wires:
  Logical Operator2/1 -> TCR Pulse Generatorr1/4(SqWave)
  TCR Pulse Generatorr/1(TCR +/-) -> TCR +/1
  BL3/1(SqWave) -> Logical Operator2/1, TCR Pulse Generatorr/4(SqWave)
  TCR Pulse Generatorr1/1(TCR +/-) -> TCR -/1
  BL3/2(Sync +) -> TCR Pulse Generatorr/3(Sync +/-)
  BL3/3(Sync -) -> TCR Pulse Generatorr1/3(Sync +/-)
  Alpha/1 -> TCR Pulse Generatorr/2(Alpha), TCR Pulse Generatorr1/2(Alpha)
  BL2/1(Ns/c) -> TCR Pulse Generatorr/1(Ns/c), TCR Pulse Generatorr1/1(Ns/c)
  "PLL sync on positive peak "/2(wt) -> Sum/2
  Sum/1 -> Trigonometric Function6/1
  Trigonometric Function6/1 -> BL3/2(sin(wt))
  Correction for delay/1 -> Sum/1
  "PLL sync on positive peak "/1(Freq) -> BL2/1(Freq), BL3/1(Freq), Correction for delay/1
  Iabc/1 -> "PLL sync on positive peak "/1(V(pu))

== system TCSC_original/Firing Unit/Firing Unit C phase ==
  note: Generate square-wave synchronised with the line current.
      | For positive (Sync +) and negative (Sync -) transition
  note: PLL
      | sync on
      | pos. peak
      | of input
  note: Generate firing
      | pulse for TCR +
  note: Generate firing
      | pulse for TCR -
  note: Compute number
      | of samples per cycle
  note: Input
      | curent
  Iabc : Inport  PortDimensions=1
  Alpha : Inport  Port=2  PortDimensions=1
  BL2 : Subsystem
  BL3 : Subsystem
  Correction for delay : Gain  Gain=Nstep*Ts*2*pi  SaturateOnIntegerOverflow=on  OutDataTypeStr=Inherit: Same as input  ParamDataTypeStr=Inherit: Same as input
  Logical Operator2 : Logic  Operator=NOT  Inputs=3
  "PLL sync on positive peak " : Subsystem  mask(Discrete 1-phase PLL){Par_Init=[PhaseInit FreqInit], ParK=[50 500], Ts=Ts}
      mask prompts: Par_Init "Initial input:[ Phase(degrees)   Frequency(Hz) ]"; ParK "Regulator gains [ Kp  Ki ]"; Ts "Sample time:"
      mask help:
      | This Phase Locked Loop (PLL) system can be used  to synchronize on a variable frequency sinusoidal signal.
      |
      | Input 1: Normalized input signal V(pu)
      mask init:
      | Kp=ParK(1);
      | Ki=ParK(2);
      | Phase_Init=Par_Init(1);
      | Finit=Par_Init(2);
  Sum : Sum  InputSameDT=on  SaturateOnIntegerOverflow=on  OutDataTypeStr=Inherit: Same as first input
  TCR Pulse Generatorr : Subsystem  mask{Ts=Ts}
      mask prompts: Ts "Sample time:"
  TCR Pulse Generatorr1 : Subsystem  mask{Ts=Ts}
      mask prompts: Ts "Sample time:"
  Trigonometric Function6 : Trigonometry
  TCR + : Outport  VectorParamsAs1DForOutWhenUnconnected=off
  TCR - : Outport  Port=2  VectorParamsAs1DForOutWhenUnconnected=off
  wires:
  Logical Operator2/1 -> TCR Pulse Generatorr1/4(SqWave)
  TCR Pulse Generatorr/1(TCR +/-) -> TCR +/1
  BL3/1(SqWave) -> Logical Operator2/1, TCR Pulse Generatorr/4(SqWave)
  TCR Pulse Generatorr1/1(TCR +/-) -> TCR -/1
  BL3/2(Sync +) -> TCR Pulse Generatorr/3(Sync +/-)
  BL3/3(Sync -) -> TCR Pulse Generatorr1/3(Sync +/-)
  Alpha/1 -> TCR Pulse Generatorr/2(Alpha), TCR Pulse Generatorr1/2(Alpha)
  BL2/1(Ns/c) -> TCR Pulse Generatorr/1(Ns/c), TCR Pulse Generatorr1/1(Ns/c)
  "PLL sync on positive peak "/2(wt) -> Sum/2
  Sum/1 -> Trigonometric Function6/1
  Trigonometric Function6/1 -> BL3/2(sin(wt))
  Correction for delay/1 -> Sum/1
  "PLL sync on positive peak "/1(Freq) -> BL2/1(Freq), BL3/1(Freq), Correction for delay/1
  Iabc/1 -> "PLL sync on positive peak "/1(V(pu))

== system TCSC_original/Firing Unit/current p.u. ==
  note: p.u current
  note: 180deg phase shift for
      | synchronisation in inductive mode
  Iabc : Inport
  alpha : Inport  Port=2
  Irms : Inport  Port=3
  Divide : Product  Inputs=*/
  Filter : Subsystem  TreatAsAtomicUnit=on
  Switch : Switch  Threshold=49  SaturateOnIntegerOverflow=off  InputSameDT=off
  delay : Gain  Gain=sqrt(2)  SaturateOnIntegerOverflow=on  OutDataTypeStr=Inherit: Same as input  ParamDataTypeStr=Inherit: Same as input
  delay1 : Gain  Gain=-1  SaturateOnIntegerOverflow=on  OutDataTypeStr=Inherit: Same as input  ParamDataTypeStr=Inherit: Same as input
  "Iabc_pu " : Outport  VectorParamsAs1DForOutWhenUnconnected=off
  wires:
  alpha/1 -> Switch/2
  Iabc/1 -> Divide/1
  Divide/1 -> "Iabc_pu "/1
  Filter/1(Out1) -> Switch/1, delay1/1
  Switch/1 -> delay/1
  delay1/1 -> Switch/3
  Irms/1 -> Filter/1(In1)
  delay/1 -> Divide/2

== system TCSC_original/Control System/Controller capacitive mode/Filter ==
  In1 : Inport
  Add : Sum  Inputs=+-
  Discrete-Time Integrator : DiscreteIntegrator  gainval=150  InitialCondition=90  SampleTime=Ts  ICPrevOutput=DiscIntNeverNeededParam  ICPrevScaledInput=DiscIntNeverNeededParam
  Out1 : Outport  VectorParamsAs1DForOutWhenUnconnected=off
  wires:
  In1/1 -> Add/1
  Discrete-Time Integrator/1 -> Out1/1, Add/2
  Add/1 -> Discrete-Time Integrator/1

== system TCSC_original/Control System/Controller inductive mode/Filter ==
  In1 : Inport
  Add : Sum  Inputs=+-
  Discrete-Time Integrator : DiscreteIntegrator  gainval=150  SampleTime=Ts  ICPrevOutput=DiscIntNeverNeededParam  ICPrevScaledInput=DiscIntNeverNeededParam
  Out1 : Outport  VectorParamsAs1DForOutWhenUnconnected=off
  wires:
  In1/1 -> Add/1
  Discrete-Time Integrator/1 -> Out1/1, Add/2
  Add/1 -> Discrete-Time Integrator/1

== system TCSC_original/Control System/Impedance calculation/RMS ==
  signal : Inport
  Abs : Abs
  Discrete-Time Integrator : DiscreteIntegrator  SampleTime=Ts  ICPrevOutput=DiscIntNeverNeededParam  ICPrevScaledInput=DiscIntNeverNeededParam
  Gain : Gain  Gain=f1  SaturateOnIntegerOverflow=on  OutDataTypeStr=Inherit: Same as input  ParamDataTypeStr=Inherit: Same as input
  Math Function : Math  Operator=square  SignedPower=on
  Math Function1 : Math  Operator=sqrt  SignedPower=on
  Sum1 : Sum  Inputs=+-  InputSameDT=on  SaturateOnIntegerOverflow=on  OutDataTypeStr=Inherit: Same as first input
  T : TransportDelay  DelayTime=1/f1
  rms : Outport  InitialOutput=0  VectorParamsAs1DForOutWhenUnconnected=off
  wires:
  Gain/1 -> Discrete-Time Integrator/1
  Math Function/1 -> Gain/1
  signal/1 -> Math Function/1
  Math Function1/1 -> rms/1
  Discrete-Time Integrator/1 -> Sum1/1, T/1
  T/1 -> Sum1/2
  Sum1/1 -> Abs/1
  Abs/1 -> Math Function1/1

== system TCSC_original/Control System/Impedance calculation/RMS1 ==
  signal : Inport
  Abs : Abs
  Discrete-Time Integrator : DiscreteIntegrator  SampleTime=Ts  ICPrevOutput=DiscIntNeverNeededParam  ICPrevScaledInput=DiscIntNeverNeededParam
  Gain : Gain  Gain=f1  SaturateOnIntegerOverflow=on  OutDataTypeStr=Inherit: Same as input  ParamDataTypeStr=Inherit: Same as input
  Math Function : Math  Operator=square  SignedPower=on
  Math Function1 : Math  Operator=sqrt  SignedPower=on
  Sum1 : Sum  Inputs=+-  InputSameDT=on  SaturateOnIntegerOverflow=on  OutDataTypeStr=Inherit: Same as first input
  T : TransportDelay  DelayTime=1/f1
  rms : Outport  InitialOutput=0  VectorParamsAs1DForOutWhenUnconnected=off
  wires:
  Gain/1 -> Discrete-Time Integrator/1
  Math Function/1 -> Gain/1
  signal/1 -> Math Function/1
  Math Function1/1 -> rms/1
  Discrete-Time Integrator/1 -> Sum1/1, T/1
  T/1 -> Sum1/2
  Sum1/1 -> Abs/1
  Abs/1 -> Math Function1/1

== system TCSC_original/Control System/Impedance calculation/RMS2 ==
  signal : Inport
  Abs : Abs
  Discrete-Time Integrator : DiscreteIntegrator  SampleTime=Ts  ICPrevOutput=DiscIntNeverNeededParam  ICPrevScaledInput=DiscIntNeverNeededParam
  Gain : Gain  Gain=f1  SaturateOnIntegerOverflow=on  OutDataTypeStr=Inherit: Same as input  ParamDataTypeStr=Inherit: Same as input
  Math Function : Math  Operator=square  SignedPower=on
  Math Function1 : Math  Operator=sqrt  SignedPower=on
  Sum1 : Sum  Inputs=+-  InputSameDT=on  SaturateOnIntegerOverflow=on  OutDataTypeStr=Inherit: Same as first input
  T : TransportDelay  DelayTime=1/f1
  rms : Outport  InitialOutput=0  VectorParamsAs1DForOutWhenUnconnected=off
  wires:
  Gain/1 -> Discrete-Time Integrator/1
  Math Function/1 -> Gain/1
  signal/1 -> Math Function/1
  Math Function1/1 -> rms/1
  Discrete-Time Integrator/1 -> Sum1/1, T/1
  T/1 -> Sum1/2
  Sum1/1 -> Abs/1
  Abs/1 -> Math Function1/1

== system TCSC_original/Control System/Impedance calculation/RMS3 ==
  signal : Inport
  Abs : Abs
  Discrete-Time Integrator : DiscreteIntegrator  SampleTime=Ts  ICPrevOutput=DiscIntNeverNeededParam  ICPrevScaledInput=DiscIntNeverNeededParam
  Gain : Gain  Gain=f1  SaturateOnIntegerOverflow=on  OutDataTypeStr=Inherit: Same as input  ParamDataTypeStr=Inherit: Same as input
  Math Function : Math  Operator=square  SignedPower=on
  Math Function1 : Math  Operator=sqrt  SignedPower=on
  Sum1 : Sum  Inputs=+-  InputSameDT=on  SaturateOnIntegerOverflow=on  OutDataTypeStr=Inherit: Same as first input
  T : TransportDelay  DelayTime=1/f1
  rms : Outport  InitialOutput=0  VectorParamsAs1DForOutWhenUnconnected=off
  wires:
  Gain/1 -> Discrete-Time Integrator/1
  Math Function/1 -> Gain/1
  signal/1 -> Math Function/1
  Math Function1/1 -> rms/1
  Discrete-Time Integrator/1 -> Sum1/1, T/1
  T/1 -> Sum1/2
  Sum1/1 -> Abs/1
  Abs/1 -> Math Function1/1

== system TCSC_original/Control System/Impedance calculation/RMS4 ==
  signal : Inport
  Abs : Abs
  Discrete-Time Integrator : DiscreteIntegrator  SampleTime=Ts  ICPrevOutput=DiscIntNeverNeededParam  ICPrevScaledInput=DiscIntNeverNeededParam
  Gain : Gain  Gain=f1  SaturateOnIntegerOverflow=on  OutDataTypeStr=Inherit: Same as input  ParamDataTypeStr=Inherit: Same as input
  Math Function : Math  Operator=square  SignedPower=on
  Math Function1 : Math  Operator=sqrt  SignedPower=on
  Sum1 : Sum  Inputs=+-  InputSameDT=on  SaturateOnIntegerOverflow=on  OutDataTypeStr=Inherit: Same as first input
  T : TransportDelay  DelayTime=1/f1
  rms : Outport  InitialOutput=0  VectorParamsAs1DForOutWhenUnconnected=off
  wires:
  Gain/1 -> Discrete-Time Integrator/1
  Math Function/1 -> Gain/1
  signal/1 -> Math Function/1
  Math Function1/1 -> rms/1
  Discrete-Time Integrator/1 -> Sum1/1, T/1
  T/1 -> Sum1/2
  Sum1/1 -> Abs/1
  Abs/1 -> Math Function1/1

== system TCSC_original/Control System/Impedance calculation/RMS5 ==
  signal : Inport
  Abs : Abs
  Discrete-Time Integrator : DiscreteIntegrator  SampleTime=Ts  ICPrevOutput=DiscIntNeverNeededParam  ICPrevScaledInput=DiscIntNeverNeededParam
  Gain : Gain  Gain=f1  SaturateOnIntegerOverflow=on  OutDataTypeStr=Inherit: Same as input  ParamDataTypeStr=Inherit: Same as input
  Math Function : Math  Operator=square  SignedPower=on
  Math Function1 : Math  Operator=sqrt  SignedPower=on
  Sum1 : Sum  Inputs=+-  InputSameDT=on  SaturateOnIntegerOverflow=on  OutDataTypeStr=Inherit: Same as first input
  T : TransportDelay  DelayTime=1/f1
  rms : Outport  InitialOutput=0  VectorParamsAs1DForOutWhenUnconnected=off
  wires:
  Gain/1 -> Discrete-Time Integrator/1
  Math Function/1 -> Gain/1
  signal/1 -> Math Function/1
  Math Function1/1 -> rms/1
  Discrete-Time Integrator/1 -> Sum1/1, T/1
  T/1 -> Sum1/2
  Sum1/1 -> Abs/1
  Abs/1 -> Math Function1/1
